simulink model "Single_Marker_Trial"  (Simulink 7.7)
settings: Solver=ode4  StartTime=0.0  StopTime=inf  FixedStep=sample_time_Vicon  RelTol=1e-3
InitFcn:
  | sample_time_Vicon = 0.005;
  | sample_time=0.02;
  | DeltaT = sample_time;
  | H0 = 0.35;
  | Kl = 1;
  | Omega_r =1.2; %1.3
  | omega_circle = 36*pi/180;
  | PI = pi;
libraries: dspadpt3 x1
settings Model: Creator=ttcl3  LastModifiedBy=Vicon
settings SolverCC: MaxConsecutiveMinStep=auto
settings OptimizationCC: EfficientMapNaN2IntZero=off
settings DebuggingCC: MultiTaskRateTransMsg=warning
settings HardwareCC: TargetIntDivRoundTo=Zero  TargetEndianess=LittleEndian  TargetHWDeviceType=MATLAB Host  ProdEqTarget=off
settings SFSimCC: SimParseCustomCode=off
settings CodeAppCC: MaxIdLength=128

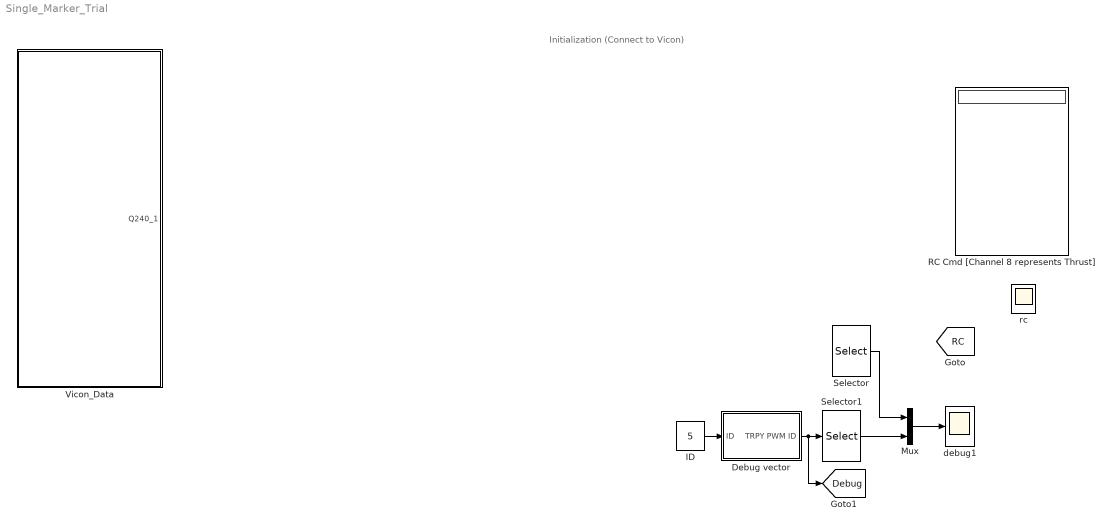
== system Single_Marker_Trial ==
  note: Initialization
      | (Connect to Vicon)
  Debug vector : Subsystem
  ID : Constant  Value=5
  Mux : Mux  Inputs=2
  RC Cmd [Channel 8 represents Thrust] : Display
  Selector : Selector  InputPortWidth=6  IndexOptions=Index vector (dialog)  Indices=[3]  OutputSizes=1
  Selector1 : Selector  InputPortWidth=6  IndexOptions=Index vector (dialog)  Indices=1  OutputSizes=1
  Vicon_Data : Subsystem
  debug1 : Scope
      settings: TimeRange=10  YMin=-1.3  YMax=1  SaveName=ScopeData2
  rc : Scope
      settings: TimeRange=10  YMin=-1  YMax=0.05
  tag scope: Debug=global, RC=global
  wires:
  ? -> RC Cmd [Channel 8 represents Thrust]/1, [RC], rc/1
  Mux/1 -> debug1/1
  Debug vector/1(TRPY PWM ID) -> Selector1/1, [Debug]
  ID/1 -> Debug vector/1(ID)
  Selector/1 -> Mux/1
  Selector1/1 -> Mux/2

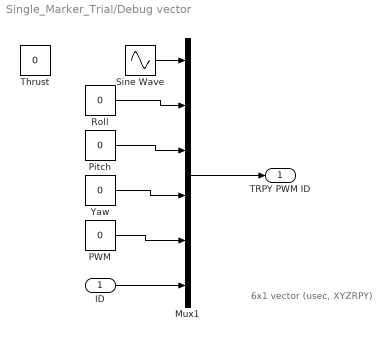
== system Single_Marker_Trial/Debug vector ==
  note: 6x1 vector (usec, XYZRPY)
  ID : Inport
  Mux1 : Mux  Inputs=6
  PWM : Constant  Value=0
  Pitch : Constant  Value=0
  Roll : Constant  Value=0
  Sine Wave : Sin  SampleTime=0
  Thrust : Constant  Value=0
  Yaw : Constant  Value=0
  TRPY PWM ID : Outport
  wires:
  Mux1/1 -> TRPY PWM ID/1
  Roll/1 -> Mux1/2
  Pitch/1 -> Mux1/3
  Yaw/1 -> Mux1/4
  PWM/1 -> Mux1/5
  ID/1 -> Mux1/6
  Sine Wave/1 -> Mux1/1

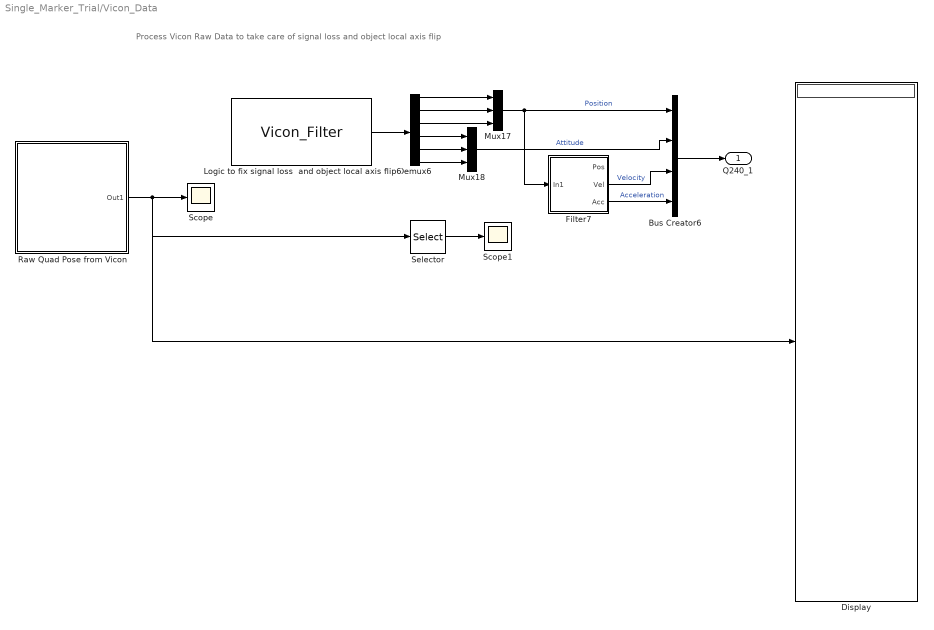
== system Single_Marker_Trial/Vicon_Data ==
  note: Process Vicon Raw Data to take care of signal loss and object local axis flip
  Bus Creator6 : BusCreator
  Demux6 : Demux  Outputs=6
  Display : Display
  Filter7 : Subsystem
  Logic to fix signal loss  and object local axis flip6 : M-S-Function  FunctionName=Vicon_Filter
  Mux17 : Mux  Inputs=3
  Mux18 : Mux  Inputs=3
  Raw Quad Pose from Vicon : Subsystem
  Scope : Scope
      settings: YMin=-800  YMax=100
  Scope1 : Scope
      settings: YMin=-5500  YMax=3500  SaveName=ScopeData3
  Selector : Selector  InputPortWidth=30  IndexOptions=Index vector (dialog)  Indices=[1 2 3 ]  OutputSizes=1
  Q240_1 : Outport
  wires:
  Logic to fix signal loss  and object local axis flip6/1 -> Demux6/1
  Demux6/1 -> Mux17/1
  Demux6/2 -> Mux17/2
  Demux6/3 -> Mux17/3
  Demux6/4 -> Mux18/1
  Demux6/5 -> Mux18/2
  Demux6/6 -> Mux18/3
  Filter7/2(Vel) -> Bus Creator6/3  "Velocity"
  Mux17/1 -> Bus Creator6/1, Filter7/1(In1)  "Position"
  Filter7/3(Acc) -> Bus Creator6/4  "Acceleration"
  Mux18/1 -> Bus Creator6/2  "Attitude"
  Bus Creator6/1 -> Q240_1/1
  Raw Quad Pose from Vicon/1(Out1) -> Display/1, Scope/1, Selector/1
  Selector/1 -> Scope1/1

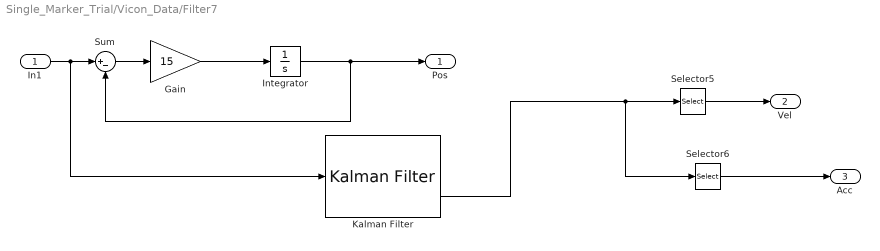
== system Single_Marker_Trial/Vicon_Data/Filter7 ==
  In1 : Inport
  Gain : Gain  Gain=15
  Integrator : Integrator
  Kalman Filter : dspadpt3/Kalman Filter  SystemSampleTime=-1  num_targets=1  sourceEnable=Always  isReset=on  X=zeros([9, 1])  P=zeros(9)  A=[1 sample_time_Vicon sample_time_Vicon*sample_time_Vicon/2 zeros(1,6);0 1 sample_time_Vicon zeros(1,6);0 0 1 zeros(1,6);0 0 0 1 sample_time_Vicon sample_time_Vicon*sample_time_Vicon/2 0 0 0;zeros(1,4) 1 sample_time_Vicon zeros(1,3);zeros(1,5) 1 zeros(1,3);zeros(1,6) 1 sample_time_Vicon sample_time_Vicon*sample_time_Vicon/2;zeros(1,7) 1 sample_time_Vicon;zeros(1,8) 1]  sourceMeasure=Specify via Dialog  H=[1 zeros(1,8); zeros(1,3) 1 zeros(1,5);zeros(1,6) 1 0 0]  Q=diag([0 0.001 0.001 0 0.001 0.001 0 0.001 0.001])  R=0.001*eye(3)  isOutputEstMeasure=on  isOutputEstState=on  isOutputEstError=off  isOutputPrdMeasure=off  isOutputPrdState=off  isOutputPrdError=off
  Selector5 : Selector  InputPortWidth=9  IndexOptions=Index vector (dialog)  Indices=[2 5 8]  OutputSizes=1
  Selector6 : Selector  InputPortWidth=9  IndexOptions=Index vector (dialog)  Indices=[3 6 9]  OutputSizes=1
  Sum : Sum  Inputs=|+-
  Pos : Outport
  Vel : Outport  Port=2
  Acc : Outport  Port=3
  wires:
  Selector6/1 -> Acc/1
  Kalman Filter/2 -> Selector6/1, Selector5/1
  In1/1 -> Sum/1, Kalman Filter/1
  Integrator/1 -> Sum/2, Pos/1
  Gain/1 -> Integrator/1
  Sum/1 -> Gain/1
  Selector5/1 -> Vel/1

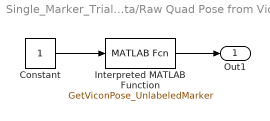
== system Single_Marker_Trial/Vicon_Data/Raw Quad Pose from Vicon ==
  Constant : Constant
  Interpreted MATLAB Function : MATLABFcn  MATLABFcn=GetViconPose_UnlabeledMarker
  Out1 : Outport
  wires:
  Constant/1 -> Interpreted MATLAB Function/1
  Interpreted MATLAB Function/1 -> Out1/1
